simulink model "Single_current_Vin_Vc_integrator_method"  (R2024a)
settings: Solver=VariableStepAuto  StartTime=0.0  StopTime=10.0  RelTol=1e-3
values from neighbouring files (symbols this model uses):
  C = 10    [Single_current_Vin_Vc_Iout_parameters.mat]
  L = 20    [Single_current_Vin_Vc_Iout_parameters.mat]
  R = 5    [Single_current_Vin_Vc_Iout_parameters.mat]
settings Model: Creator=nassa  LastModifiedBy=nassa

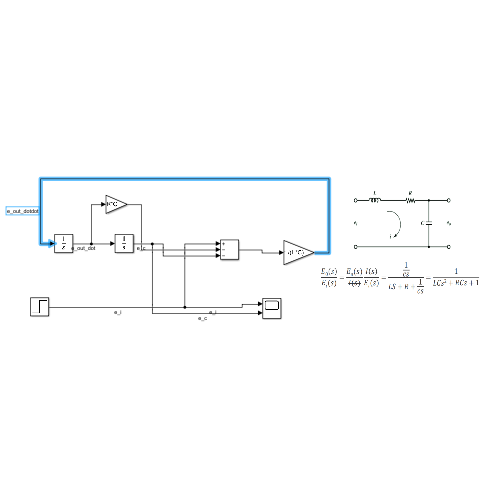
[thumbnail: Simulink's stored preview of the top-level diagram]
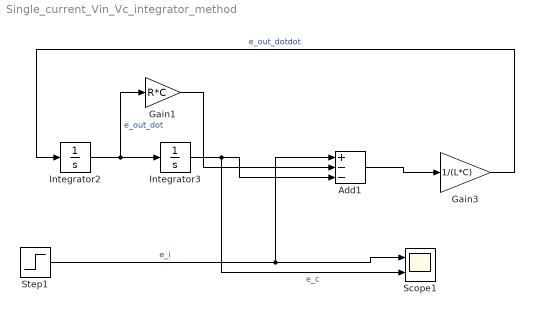
== system Single_current_Vin_Vc_integrator_method ==
  Add1 : Sum  Inputs=+--
  Gain1 : Gain  Gain=R*C
  Gain3 : Gain  Gain=1/(L*C)
  Integrator2 : Integrator
  Integrator3 : Integrator
  Scope1 : Scope  NumInputPorts=2
  Step1 : Step  SampleTime=0
  wires:
  Integrator3/1 -> Scope1/2, Add1/3  "e_c"
  Integrator2/1 -> Gain1/1, Integrator3/1  "e_out_dot"
  Step1/1 -> Scope1/1, Add1/1  "e_i"
  Gain1/1 -> Add1/2
  Gain3/1 -> Integrator2/1  "e_out_dotdot"
  Add1/1 -> Gain3/1
